simulink model "paneltest"  (R2017a)
settings: Solver=ode45  StartTime=0.0  StopTime=10  RelTol=1e-3
libraries: powerlib x2, powerlib_extras x1, re_lib x1
settings Model: Creator=acer  LastModifiedBy=acer

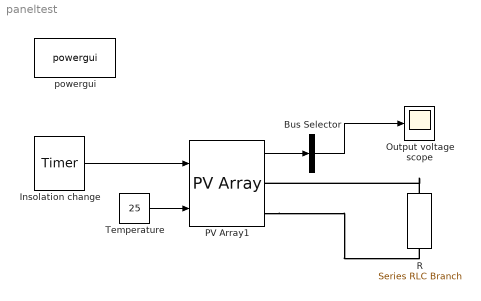
== system paneltest ==
  Bus Selector : BusSelector  OutputSignals=V_PV  OutputAsBus=on
  Insolation change : powerlib_extras/Control  Blocks/Timer  t="[0  5]"  e=[1000 800]
  Output voltage scope : Scope
  PV Array1 : re_lib/Solar/PV Array  Npar=4  Nser=9  PlotType=one module @ 25 deg.C & specified irradiances  S_vec=[1000 800]  Temp_C_vec="[ 45 25  ]"  ModuleName=User-defined  PlotWhenSelected=on  Pm=20.1544  Ncell=36  Voc=21.17  Isc=1.26  Vm=17.08  Im=1.18  beta_Voc_pc=-0.2941  alpha_Isc_pc=0.0681  beta_Voc=-0.062261  alpha_Isc=0.00085806  IL=1.2621  I0=3.4157e-12  nI=0.85997  Rsh=849.2491  Rs=1.4265  BAL=on  Tc=1e-6  Tfilter=2e-5
  R : powerlib/Elements/Series RLC Branch  LConnTagsString=__new0  RConnTagsString=__new0  BranchType=R  Resistance=3.5  Inductance=1e-3  SetiL0=off  InitialCurrent=0  Capacitance=1e-6  Setx0=off  InitialVoltage=0  Measurements=None
  Temperature : Constant  Value=25  VectorParams1D=off  SampleTime=.05
  powergui : powerlib/powergui  Priority=1  SimulationMode=Discrete  SampleTime=50e-6  frequency=60  Iterations=50  frequencyindice=0  Pbase=100e6  ErrMax=1e-4  UnitsV=kV  UnitsW=MW  buscounter=0  FunctionMessages=off  echomessages=off  EnableUseOfTLC=off  CurrentSourceSwitches=off  DisableSnubberDevices=off  DisableRonSwitches=off  DisableVfSwitches=off  DisplayEquations=off  SolverType=Tustin/Backward Euler (TBE)  Interpol=off  ExternalGateDelay=off  methode=off  Ts=100  x0status=blocks  SPID=on  SwTol=0  HookPort=off  RestoreLinks=warning  ResistiveCurrentMeasurement=off  Frange=[0:2:500]  Ylog=off  Xlog=on  ShowGrid=off  save=off  variable=ZData  structure=0  ZoomFFT=off  StartTime=0.0  cycles=1  DisplayStyle=1  fundamental=60  FreqAxis=off  MaxFrequency=1000  frequencyindicesteady=1  RmsSteady=1  display=off
  wires:
  Insolation change/1 -> PV Array1/1
  Temperature/1 -> PV Array1/2
  PV Array1/1 -> Bus Selector/1
  Bus Selector/1 -> Output voltage scope/1
  connections:
  R/LConn1 -- PV Array1/RConn1
  PV Array1/RConn2 -- R/RConn1
